simulink library "Components"  (R2023b)
settings: Solver=VariableStepAuto  StartTime=0.0  StopTime=10.0  RelTol=1e-3
undefined symbols (not defined in the file): BIT_MASK_010_CENTS, BIT_MASK_020_CENTS, BIT_MASK_050_CENTS, BIT_MASK_100_CENTS, BIT_MASK_200_CENTS, char2dec
libraries: simulink x6
Description:
  | % Copyright 2023 The MathWorks, Inc.
settings Model: Creator=sdupertu  LastModifiedBy=sebas
settings SolverCC: AlgebraicLoopSolver=TrustRegion
settings DebuggingCC: UnconnectedInputMsg=warning  UnconnectedOutputMsg=warning  UnconnectedLineMsg=warning  PregeneratedLibrarySubsystemCodeDiagnostic=none  ArithmeticOperatorsInVariantConditions=warning
settings ModelReferenceCC: EnableRefExpFcnMdlSchedulingChecks=on
settings SFSimCC: SimUseLocalCustomCode=off  CustomCodeUndefinedFunction=UseInterfaceOnly
settings RTWCC: RTWUseLocalCustomCode=off  DLArmComputeVersion=19.05

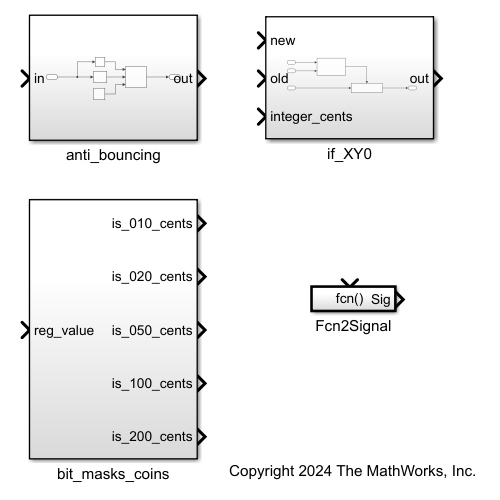
[thumbnail: Simulink's stored preview of the top-level diagram]
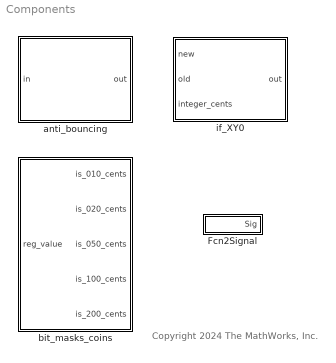
== system Components ==
  note: Copyright 2024 The MathWorks, Inc.
  Fcn2Signal : Subsystem
  anti_bouncing : Subsystem
  bit_masks_coins : Subsystem
  if_XY0 : Subsystem

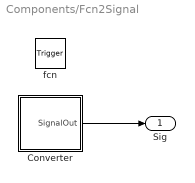
== system Components/Fcn2Signal ==
  fcn : TriggerPort  TriggerType=function-call  VariantControl=Variant  SampleTime=-1
  Converter : Stateflow chart  BlockKeywords=__PRM__SERIALIZED__DATA__:Stateflow Chart,Stateflow Diagram  TreatAsAtomicUnit=on
  Sig : Outport  OutDataTypeStr=boolean  InitialOutput=false  VectorParamsAs1DForOutWhenUnconnected=off
  wires:
  Converter/1(SignalOut) -> Sig/1

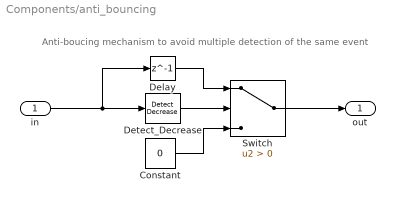
== system Components/anti_bouncing ==
  note: Anti-boucing mechanism to avoid multiple detection of the same event
  in : Inport
  Constant : Constant  Value=0  OutDataTypeStr=uint8  SampleTime=-1
  Delay : Delay  DelayLength=1  InitialCondition=0
  Detect_Decrease : simulink/Logic and Bit Operations/Detect Decrease  vinit=0  OutDataTypeStr=uint8
  Switch : Switch  Criteria=u2 > Threshold  SaturateOnIntegerOverflow=off  InputSameDT=off
  out : Outport  VectorParamsAs1DForOutWhenUnconnected=off
  wires:
  in/1 -> Delay/1, Detect_Decrease/1
  Switch/1 -> out/1
  Constant/1 -> Switch/3
  Delay/1 -> Switch/1
  Detect_Decrease/1 -> Switch/2

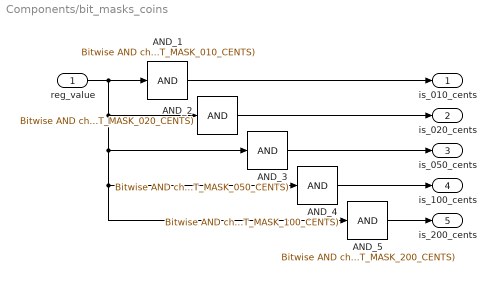
== system Components/bit_masks_coins ==
  reg_value : Inport
  AND_1 : simulink/Logic and Bit Operations/Bitwise Operator  logicop=AND  UseBitMask=on  BitMask=char2dec(BIT_MASK_010_CENTS)  BitMaskRealWorld=Stored Integer
  AND_2 : simulink/Logic and Bit Operations/Bitwise Operator  logicop=AND  UseBitMask=on  BitMask=char2dec(BIT_MASK_020_CENTS)  BitMaskRealWorld=Stored Integer
  AND_3 : simulink/Logic and Bit Operations/Bitwise Operator  logicop=AND  UseBitMask=on  BitMask=char2dec(BIT_MASK_050_CENTS)  BitMaskRealWorld=Stored Integer
  AND_4 : simulink/Logic and Bit Operations/Bitwise Operator  logicop=AND  UseBitMask=on  BitMask=char2dec(BIT_MASK_100_CENTS)  BitMaskRealWorld=Stored Integer
  AND_5 : simulink/Logic and Bit Operations/Bitwise Operator  logicop=AND  UseBitMask=on  BitMask=char2dec(BIT_MASK_200_CENTS)  BitMaskRealWorld=Stored Integer
  is_010_cents : Outport  VectorParamsAs1DForOutWhenUnconnected=off
  is_020_cents : Outport  Port=2  VectorParamsAs1DForOutWhenUnconnected=off
  is_050_cents : Outport  Port=3  VectorParamsAs1DForOutWhenUnconnected=off
  is_100_cents : Outport  Port=4  VectorParamsAs1DForOutWhenUnconnected=off
  is_200_cents : Outport  Port=5  VectorParamsAs1DForOutWhenUnconnected=off
  wires:
  AND_2/1 -> is_020_cents/1
  AND_3/1 -> is_050_cents/1
  AND_4/1 -> is_100_cents/1
  AND_5/1 -> is_200_cents/1
  reg_value/1 -> AND_5/1, AND_4/1, AND_3/1, AND_2/1, AND_1/1
  AND_1/1 -> is_010_cents/1

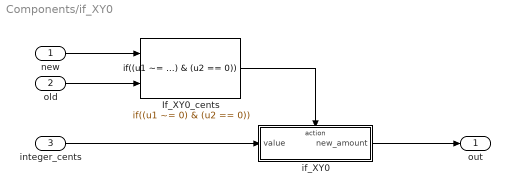
== system Components/if_XY0 ==
  new : Inport
  old : Inport  Port=2
  integer_cents : Inport  Port=3
  If_XY0_cents : If  NumInputs=2  IfExpression=(u1 ~= 0) & (u2 == 0)  ShowElse=off
  if_XY0 : Subsystem  TreatAsAtomicUnit=on
  out : Outport  VectorParamsAs1DForOutWhenUnconnected=off
  wires:
  if_XY0/1(new_amount) -> out/1
  If_XY0_cents/1 -> if_XY0/Action
  new/1 -> If_XY0_cents/1
  old/1 -> If_XY0_cents/2
  integer_cents/1 -> if_XY0/1(value)

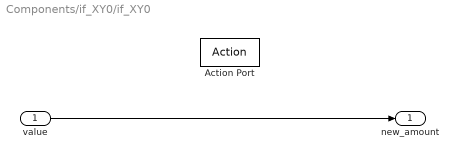
== system Components/if_XY0/if_XY0 ==
  value : Inport
  Action Port : ActionPort
  new_amount : Outport  VectorParamsAs1DForOutWhenUnconnected=off
  wires:
  value/1 -> new_amount/1

== stateflow chart Components/Fcn2Signal/Converter ==
  state Up
    entry:
    SignalOut = true;
  state Down
    entry:
    SignalOut = false;
  (default) -> Up
  Up -> Down
  Down -> Up
  data: SignalOut output boolean
